simulink model "UR5_simulink"  (R2022b)
settings: Solver=FixedStepAuto  StartTime=0.0  StopTime=8  FixedStep=1e-4  RelTol=1e-3  AbsTol=1e-3  EnableMultiTasking=on
values from neighbouring files (symbols this model uses):
  a1 = 0    [UR5_matlab.m]
  a2 = -0.425    [UR5_matlab.m]
  a3 = -0.39225    [UR5_matlab.m]
  a4 = 0    [UR5_matlab.m]
  a5 = 0    [UR5_matlab.m]
  a6 = 0    [UR5_matlab.m]
  d1 = 0.089159    [UR5_matlab.m]
  d2 = 0    [UR5_matlab.m]
  d3 = 0    [UR5_matlab.m]
  d4 = 0.10915    [UR5_matlab.m]
  d5 = 0.09465    [UR5_matlab.m]
  d6 = 0.0823    [UR5_matlab.m]
  K_fb_1 = fb_action(K1_20,N,Jin_20,Bmw,J1_est,wR1)    [UR5_matlab.m]
  K_fb_2 = fb_action(K1_20,N,Jin_20,Bmw,J2_est,wR2)    [UR5_matlab.m]
  K_fb_3 = fb_action(K1_20,N,Jin_20,Bmw,J3_est,wR3)    [UR5_matlab.m]
  K_fb_4 = fb_action(K1_14,N,Jin_14,Bmw,J4_est,wR4)    [UR5_matlab.m]
  K_fb_5 = fb_action(K1_14,N,Jin_14,Bmw,J5_est,wR5)    [UR5_matlab.m]
  K_fb_6 = fb_action(K1_14,N,Jin_14,Bmw,J6_est,wR6)    [UR5_matlab.m]
  m1 = 3.7    [UR5_matlab.m]
  m2 = 8.393    [UR5_matlab.m]
  m3 = 2.33    [UR5_matlab.m]
  m4 = 1.1219    [UR5_matlab.m]
  m5 = 1.1219    [UR5_matlab.m]
  m6 = 0.1879    [UR5_matlab.m]
  N = 100    [UR5_matlab.m]
undefined symbols (not defined in the file or in its folder): X, Y, Z
libraries: fl_lib x60, sm_lib x33, nesl_utility x31, MyComponent_lib x12
(part 2 of 2)

== system UR5_simulink/Joint 1 ==
  PS-Simulink Converter1 : nesl_utility/PS-Simulink Converter  PhysicalDomain=network_engine_domain  SubClassName=ps_output  LeftPortType=input  RightPortType=output  PseudoPeriodic=off  Frequencies=[]  VectorFormat=1-D array  Unit=inherit  AffineConversion=off
  PS-Simulink Converter2 : nesl_utility/PS-Simulink Converter  PhysicalDomain=network_engine_domain  SubClassName=ps_output  LeftPortType=input  RightPortType=output  PseudoPeriodic=off  Frequencies=[]  VectorFormat=1-D array  Unit=inherit  AffineConversion=off
  R(x1,apha1) : sm_lib/Frames and Transforms/Rigid Transform  TranslationMethod=None  TranslationStandardOffset=0  TranslationLengthUnit=m  TranslationStandardAxis=+Z  TranslationCartesianOffset=[0 0 0]  TranslationROffset=0  TranslationROffsetUnits=m  TranslationZOffset=0  TranslationZOffsetUnits=m  TranslationThetaOffset=0  TranslationThetaOffsetUnits=deg  RotationMethod=StandardAxis  RotationAngleUnits=deg  RotationStandardAxis=+X  RotationAngle=alpha1  RotationArbitraryAxis=[0 0 1]  FollAlignAxisA=+X  BaseAlignAxisA=+Y  FollAlignAxisB=+Y  BaseAlignAxisB=+Z  RotationSequenceAxes=FollowerAxes  RotationSequence=XYX  RotationSequenceAngles=[0 0 0]  RotationSequenceAnglesUnits=deg  RotationMatrix=|  Quaternion=[1 0 0 0]
      | [1 0 0; 0 0 -1;
      | 0 1 0]
  R(zo,q1) : sm_lib/Joints/Revolute Joint  JointMode=Normal  SenseConstraintForce=off  SenseConstraintForceX=off  SenseConstraintForceY=off  SenseConstraintForceZ=off  SenseConstraintTorque=off  SenseConstraintTorqueX=off  SenseConstraintTorqueY=off  SenseConstraintTorqueZ=off  SenseTotalForce=off  SenseTotalForceX=off  SenseTotalForceY=off  SenseTotalForceZ=off  SenseTotalTorque=off  SenseTotalTorqueX=off  SenseTotalTorqueY=off  SenseTotalTorqueZ=off  CompositeWrenchDir=FollowerOnBase  CompositeWrenchFrame=BaseFrame  EquilibriumPosition=0  EquilibriumPositionUnits=deg  SpringStiffness=0  SpringStiffnessUnits=N*m/deg  DampingCoefficient=0  DampingCoefficientUnits=N*m/(deg/s)  TorqueActuationMode=InputTorque  MotionActuationMode=ComputedMotion  SensePosition=on  SenseVelocity=on  SenseAcceleration=off  SenseTorqueForce=off  SenseLowerLimitTorqueForce=off  SenseUpperLimitTorqueForce=off  LowerLimitSpecify=off  LowerLimitBound=-90  LowerLimitBoundUnits=deg  LowerLimitStiffness=1e4  LowerLimitStiffnessUnits=N*m/deg  LowerLimitDamping=10  LowerLimitDampingUnits=N*m/(deg/s)  LowerLimitTransitionRegionWidth=0.1  LowerLimitTransitionRegionWidthUnits=deg  UpperLimitSpecify=off  UpperLimitBound=90  UpperLimitBoundUnits=deg  UpperLimitStiffness=1e4  UpperLimitStiffnessUnits=N*m/deg  UpperLimitDamping=10  UpperLimitDampingUnits=N*m/(deg/s)  UpperLimitTransitionRegionWidth=0.1  UpperLimitTransitionRegionWidthUnits=deg  PositionTargetSpecify=off  PositionTargetPriority=High  PositionTargetValue=0  PositionTargetValueUnits=deg  VelocityTargetSpecify=off  VelocityTargetPriority=High  VelocityTargetValue=0  VelocityTargetValueUnits=deg/s
  T(x1,a1) : sm_lib/Frames and Transforms/Rigid Transform  TranslationMethod=Cartesian  TranslationStandardOffset=0  TranslationLengthUnit=m  TranslationStandardAxis=+X  TranslationCartesianOffset=[a1 0 0]  TranslationROffset=0  TranslationROffsetUnits=m  TranslationZOffset=0  TranslationZOffsetUnits=m  TranslationThetaOffset=0  TranslationThetaOffsetUnits=deg  RotationMethod=None  RotationAngleUnits=deg  RotationStandardAxis=+Z  RotationAngle=0.0  RotationArbitraryAxis=[0 0 1]  FollAlignAxisA=+X  BaseAlignAxisA=+Y  FollAlignAxisB=+Y  BaseAlignAxisB=+Z  RotationSequenceAxes=FollowerAxes  RotationSequence=XYX  RotationSequenceAngles=[0 0 0]  RotationSequenceAnglesUnits=deg  RotationMatrix=[1 0 0; 0 1 0; 0 0 1]  Quaternion=[1 0 0 0]
  T(z0,d1) : sm_lib/Frames and Transforms/Rigid Transform  TranslationMethod=Cartesian  TranslationStandardOffset=0.089159  TranslationLengthUnit=m  TranslationStandardAxis=+Z  TranslationCartesianOffset=[0 0 d1]  TranslationROffset=0  TranslationROffsetUnits=m  TranslationZOffset=0  TranslationZOffsetUnits=m  TranslationThetaOffset=0  TranslationThetaOffsetUnits=deg  RotationMethod=None  RotationAngleUnits=deg  RotationStandardAxis=+Z  RotationAngle=0.0  RotationArbitraryAxis=[0 0 1]  FollAlignAxisA=+X  BaseAlignAxisA=+Y  FollAlignAxisB=+Y  BaseAlignAxisB=+Z  RotationSequenceAxes=FollowerAxes  RotationSequence=XYX  RotationSequenceAngles=[0 0 0]  RotationSequenceAnglesUnits=deg  RotationMatrix=[1 0 0; 0 1 0; 0 0 1]  Quaternion=[1 0 0 0]
  Link 0 : PMIOPort  Side=Left
  Link 1 : PMIOPort  Port=2  Side=Right
  Joint velocity : PMIOPort  Port=3  Side=Right
  Joint torque1 : PMIOPort  Port=4  Side=Left
  tag scope: dq1=global, q1=global
  wires:
  PS-Simulink Converter1/1 -> [q1]
  PS-Simulink Converter2/1 -> [dq1]
  connections:
  PS-Simulink Converter2/LConn1 -- R(zo,q1)/RConn3 -- Joint velocity/RConn1
  PS-Simulink Converter1/LConn1 -- R(zo,q1)/RConn2
  T(z0,d1)/LConn1 -- Link 0/RConn1
  R(zo,q1)/LConn1 -- T(z0,d1)/RConn1
  T(x1,a1)/LConn1 -- R(zo,q1)/RConn1
  Joint torque1/RConn1 -- R(zo,q1)/LConn2
  R(x1,apha1)/LConn1 -- T(x1,a1)/RConn1
  R(x1,apha1)/RConn1 -- Link 1/RConn1

== system UR5_simulink/Joint 2 ==
  PS-Simulink Converter1 : nesl_utility/PS-Simulink Converter  PhysicalDomain=network_engine_domain  SubClassName=ps_output  LeftPortType=input  RightPortType=output  PseudoPeriodic=off  Frequencies=[]  VectorFormat=1-D array  Unit=inherit  AffineConversion=off
  PS-Simulink Converter2 : nesl_utility/PS-Simulink Converter  PhysicalDomain=network_engine_domain  SubClassName=ps_output  LeftPortType=input  RightPortType=output  PseudoPeriodic=off  Frequencies=[]  VectorFormat=1-D array  Unit=inherit  AffineConversion=off
  R(x2,alpha2) : sm_lib/Frames and Transforms/Rigid Transform  TranslationMethod=None  TranslationStandardOffset=0  TranslationLengthUnit=m  TranslationStandardAxis=+Z  TranslationCartesianOffset=[-0.425 0 0]  TranslationROffset=0  TranslationROffsetUnits=m  TranslationZOffset=0  TranslationZOffsetUnits=m  TranslationThetaOffset=0  TranslationThetaOffsetUnits=deg  RotationMethod=StandardAxis  RotationAngleUnits=deg  RotationStandardAxis=+X  RotationAngle=alpha2  RotationArbitraryAxis=[0 0 1]  FollAlignAxisA=+X  BaseAlignAxisA=+Y  FollAlignAxisB=+Y  BaseAlignAxisB=+Z  RotationSequenceAxes=FollowerAxes  RotationSequence=XYX  RotationSequenceAngles=[0 0 0]  RotationSequenceAnglesUnits=deg  RotationMatrix=[1 0 0; 0 1 0; 0 0 1]  Quaternion=[1 0 0 0]
  R(z1,q2) : sm_lib/Joints/Revolute Joint  JointMode=Normal  SenseConstraintForce=off  SenseConstraintForceX=off  SenseConstraintForceY=off  SenseConstraintForceZ=off  SenseConstraintTorque=off  SenseConstraintTorqueX=off  SenseConstraintTorqueY=off  SenseConstraintTorqueZ=off  SenseTotalForce=off  SenseTotalForceX=off  SenseTotalForceY=off  SenseTotalForceZ=off  SenseTotalTorque=off  SenseTotalTorqueX=off  SenseTotalTorqueY=off  SenseTotalTorqueZ=off  CompositeWrenchDir=FollowerOnBase  CompositeWrenchFrame=BaseFrame  EquilibriumPosition=0  EquilibriumPositionUnits=deg  SpringStiffness=0  SpringStiffnessUnits=N*m/deg  DampingCoefficient=0  DampingCoefficientUnits=N*m/(deg/s)  TorqueActuationMode=InputTorque  MotionActuationMode=ComputedMotion  SensePosition=on  SenseVelocity=on  SenseAcceleration=off  SenseTorqueForce=off  SenseLowerLimitTorqueForce=off  SenseUpperLimitTorqueForce=off  LowerLimitSpecify=off  LowerLimitBound=-360  LowerLimitBoundUnits=deg  LowerLimitStiffness=1e4  LowerLimitStiffnessUnits=N*m/deg  LowerLimitDamping=10  LowerLimitDampingUnits=N*m/(deg/s)  LowerLimitTransitionRegionWidth=0.1  LowerLimitTransitionRegionWidthUnits=deg  UpperLimitSpecify=off  UpperLimitBound=360  UpperLimitBoundUnits=deg  UpperLimitStiffness=1e4  UpperLimitStiffnessUnits=N*m/deg  UpperLimitDamping=10  UpperLimitDampingUnits=N*m/(deg/s)  UpperLimitTransitionRegionWidth=0.1  UpperLimitTransitionRegionWidthUnits=deg  PositionTargetSpecify=off  PositionTargetPriority=High  PositionTargetValue=0  PositionTargetValueUnits=deg  VelocityTargetSpecify=off  VelocityTargetPriority=High  VelocityTargetValue=0  VelocityTargetValueUnits=deg/s
  T(x2,a2) : sm_lib/Frames and Transforms/Rigid Transform  TranslationMethod=Cartesian  TranslationStandardOffset=0.425  TranslationLengthUnit=m  TranslationStandardAxis=-X  TranslationCartesianOffset=[a2 0 0]  TranslationROffset=0  TranslationROffsetUnits=m  TranslationZOffset=0  TranslationZOffsetUnits=m  TranslationThetaOffset=0  TranslationThetaOffsetUnits=deg  RotationMethod=None  RotationAngleUnits=deg  RotationStandardAxis=+Z  RotationAngle=0.0  RotationArbitraryAxis=[0 0 1]  FollAlignAxisA=+X  BaseAlignAxisA=+Y  FollAlignAxisB=+Y  BaseAlignAxisB=+Z  RotationSequenceAxes=FollowerAxes  RotationSequence=XYX  RotationSequenceAngles=[0 0 0]  RotationSequenceAnglesUnits=deg  RotationMatrix=[1 0 0; 0 1 0; 0 0 1]  Quaternion=[1 0 0 0]
  T(z1,d2) : sm_lib/Frames and Transforms/Rigid Transform  TranslationMethod=Cartesian  TranslationStandardOffset=0  TranslationLengthUnit=m  TranslationStandardAxis=+Z  TranslationCartesianOffset=[0 0 d2]  TranslationROffset=0  TranslationROffsetUnits=m  TranslationZOffset=0  TranslationZOffsetUnits=m  TranslationThetaOffset=0  TranslationThetaOffsetUnits=deg  RotationMethod=None  RotationAngleUnits=deg  RotationStandardAxis=+Z  RotationAngle=0.0  RotationArbitraryAxis=[0 0 1]  FollAlignAxisA=+X  BaseAlignAxisA=+Y  FollAlignAxisB=+Y  BaseAlignAxisB=+Z  RotationSequenceAxes=FollowerAxes  RotationSequence=XYX  RotationSequenceAngles=[0 0 0]  RotationSequenceAnglesUnits=deg  RotationMatrix=[1 -0 0; 0 1 0; 0 0 1]  Quaternion=[1 0 0 0]
  Link 1 : PMIOPort  Side=Left
  "Joint torque " : PMIOPort  Port=2  Side=Left
  Link 2 : PMIOPort  Port=3  Side=Right
  Joint velocity : PMIOPort  Port=4  Side=Right
  tag scope: dq2=global, q2=global
  wires:
  PS-Simulink Converter2/1 -> [dq2]
  PS-Simulink Converter1/1 -> [q2]
  connections:
  R(z1,q2)/LConn1 -- T(z1,d2)/RConn1
  PS-Simulink Converter2/LConn1 -- R(z1,q2)/RConn3 -- Joint velocity/RConn1
  PS-Simulink Converter1/LConn1 -- R(z1,q2)/RConn2
  T(z1,d2)/LConn1 -- Link 1/RConn1
  T(x2,a2)/LConn1 -- R(z1,q2)/RConn1
  "Joint torque "/RConn1 -- R(z1,q2)/LConn2
  R(x2,alpha2)/LConn1 -- T(x2,a2)/RConn1
  Link 2/RConn1 -- R(x2,alpha2)/RConn1

== system UR5_simulink/Joint 3 ==
  PS-Simulink Converter1 : nesl_utility/PS-Simulink Converter  PhysicalDomain=network_engine_domain  SubClassName=ps_output  LeftPortType=input  RightPortType=output  PseudoPeriodic=off  Frequencies=[]  VectorFormat=1-D array  Unit=inherit  AffineConversion=off
  PS-Simulink Converter2 : nesl_utility/PS-Simulink Converter  PhysicalDomain=network_engine_domain  SubClassName=ps_output  LeftPortType=input  RightPortType=output  PseudoPeriodic=off  Frequencies=[]  VectorFormat=1-D array  Unit=inherit  AffineConversion=off
  R(x3,alpha3) : sm_lib/Frames and Transforms/Rigid Transform  TranslationMethod=None  TranslationStandardOffset=0  TranslationLengthUnit=m  TranslationStandardAxis=+Z  TranslationCartesianOffset=[-0.425 0 0]  TranslationROffset=0  TranslationROffsetUnits=m  TranslationZOffset=0  TranslationZOffsetUnits=m  TranslationThetaOffset=0  TranslationThetaOffsetUnits=deg  RotationMethod=StandardAxis  RotationAngleUnits=deg  RotationStandardAxis=+X  RotationAngle=alpha3  RotationArbitraryAxis=[0 0 1]  FollAlignAxisA=+X  BaseAlignAxisA=+Y  FollAlignAxisB=+Y  BaseAlignAxisB=+Z  RotationSequenceAxes=FollowerAxes  RotationSequence=XYX  RotationSequenceAngles=[0 0 0]  RotationSequenceAnglesUnits=deg  RotationMatrix=[1 0 0; 0 1 0; 0 0 1]  Quaternion=[1 0 0 0]
  R(z2,q3) : sm_lib/Joints/Revolute Joint  JointMode=Normal  SenseConstraintForce=off  SenseConstraintForceX=off  SenseConstraintForceY=off  SenseConstraintForceZ=off  SenseConstraintTorque=off  SenseConstraintTorqueX=off  SenseConstraintTorqueY=off  SenseConstraintTorqueZ=off  SenseTotalForce=off  SenseTotalForceX=off  SenseTotalForceY=off  SenseTotalForceZ=off  SenseTotalTorque=off  SenseTotalTorqueX=off  SenseTotalTorqueY=off  SenseTotalTorqueZ=off  CompositeWrenchDir=FollowerOnBase  CompositeWrenchFrame=BaseFrame  EquilibriumPosition=0  EquilibriumPositionUnits=deg  SpringStiffness=0  SpringStiffnessUnits=N*m/deg  DampingCoefficient=0  DampingCoefficientUnits=N*m/(deg/s)  TorqueActuationMode=InputTorque  MotionActuationMode=ComputedMotion  SensePosition=on  SenseVelocity=on  SenseAcceleration=off  SenseTorqueForce=off  SenseLowerLimitTorqueForce=off  SenseUpperLimitTorqueForce=off  LowerLimitSpecify=off  LowerLimitBound=-360  LowerLimitBoundUnits=deg  LowerLimitStiffness=1e4  LowerLimitStiffnessUnits=N*m/deg  LowerLimitDamping=10  LowerLimitDampingUnits=N*m/(deg/s)  LowerLimitTransitionRegionWidth=0.1  LowerLimitTransitionRegionWidthUnits=deg  UpperLimitSpecify=off  UpperLimitBound=360  UpperLimitBoundUnits=deg  UpperLimitStiffness=1e4  UpperLimitStiffnessUnits=N*m/deg  UpperLimitDamping=10  UpperLimitDampingUnits=N*m/(deg/s)  UpperLimitTransitionRegionWidth=0.1  UpperLimitTransitionRegionWidthUnits=deg  PositionTargetSpecify=off  PositionTargetPriority=High  PositionTargetValue=0  PositionTargetValueUnits=deg  VelocityTargetSpecify=off  VelocityTargetPriority=High  VelocityTargetValue=0  VelocityTargetValueUnits=deg/s
  T(x3,a3) : sm_lib/Frames and Transforms/Rigid Transform  TranslationMethod=Cartesian  TranslationStandardOffset=-0.39225  TranslationLengthUnit=m  TranslationStandardAxis=+X  TranslationCartesianOffset=[a3 0 0]  TranslationROffset=0  TranslationROffsetUnits=m  TranslationZOffset=0  TranslationZOffsetUnits=m  TranslationThetaOffset=0  TranslationThetaOffsetUnits=deg  RotationMethod=None  RotationAngleUnits=deg  RotationStandardAxis=+Z  RotationAngle=0.0  RotationArbitraryAxis=[0 0 1]  FollAlignAxisA=+X  BaseAlignAxisA=+Y  FollAlignAxisB=+Y  BaseAlignAxisB=+Z  RotationSequenceAxes=FollowerAxes  RotationSequence=XYX  RotationSequenceAngles=[0 0 0]  RotationSequenceAnglesUnits=deg  RotationMatrix=[1 0 0; 0 1 0; 0 0 1]  Quaternion=[1 0 0 0]
  T(z2,d3) : sm_lib/Frames and Transforms/Rigid Transform  TranslationMethod=Cartesian  TranslationStandardOffset=0  TranslationLengthUnit=m  TranslationStandardAxis=+Z  TranslationCartesianOffset=[0 0 d3]  TranslationROffset=0  TranslationROffsetUnits=m  TranslationZOffset=0  TranslationZOffsetUnits=m  TranslationThetaOffset=0  TranslationThetaOffsetUnits=deg  RotationMethod=None  RotationAngleUnits=deg  RotationStandardAxis=+Z  RotationAngle=0.0  RotationArbitraryAxis=[0 0 1]  FollAlignAxisA=+X  BaseAlignAxisA=+Y  FollAlignAxisB=+Y  BaseAlignAxisB=+Z  RotationSequenceAxes=FollowerAxes  RotationSequence=XYX  RotationSequenceAngles=[0 0 0]  RotationSequenceAnglesUnits=deg  RotationMatrix=[1 -0 0; 0 1 0; 0 0 1]  Quaternion=[1 0 0 0]
  Link 2 : PMIOPort  Side=Left
  "Joint torque " : PMIOPort  Port=2  Side=Left
  Link 3 : PMIOPort  Port=3  Side=Right
  Joint velocity : PMIOPort  Port=4  Side=Right
  tag scope: dq3=global, q3=global
  wires:
  PS-Simulink Converter2/1 -> [dq3]
  PS-Simulink Converter1/1 -> [q3]
  connections:
  PS-Simulink Converter2/LConn1 -- Joint velocity/RConn1 -- R(z2,q3)/RConn3
  PS-Simulink Converter1/LConn1 -- R(z2,q3)/RConn2
  T(z2,d3)/RConn1 -- R(z2,q3)/LConn1
  T(z2,d3)/LConn1 -- Link 2/RConn1
  T(x3,a3)/LConn1 -- R(z2,q3)/RConn1
  R(z2,q3)/LConn2 -- "Joint torque "/RConn1
  R(x3,alpha3)/RConn1 -- Link 3/RConn1
  T(x3,a3)/RConn1 -- R(x3,alpha3)/LConn1

== system UR5_simulink/Joint 4 ==
  PS-Simulink Converter1 : nesl_utility/PS-Simulink Converter  PhysicalDomain=network_engine_domain  SubClassName=ps_output  LeftPortType=input  RightPortType=output  PseudoPeriodic=off  Frequencies=[]  VectorFormat=1-D array  Unit=inherit  AffineConversion=off
  PS-Simulink Converter2 : nesl_utility/PS-Simulink Converter  PhysicalDomain=network_engine_domain  SubClassName=ps_output  LeftPortType=input  RightPortType=output  PseudoPeriodic=off  Frequencies=[]  VectorFormat=1-D array  Unit=inherit  AffineConversion=off
  R(x4,alpha4) : sm_lib/Frames and Transforms/Rigid Transform  TranslationMethod=None  TranslationStandardOffset=0  TranslationLengthUnit=m  TranslationStandardAxis=+Z  TranslationCartesianOffset=[0 0 0]  TranslationROffset=0  TranslationROffsetUnits=m  TranslationZOffset=0  TranslationZOffsetUnits=m  TranslationThetaOffset=0  TranslationThetaOffsetUnits=deg  RotationMethod=StandardAxis  RotationAngleUnits=deg  RotationStandardAxis=+X  RotationAngle=alpha4  RotationArbitraryAxis=[0 0 1]  FollAlignAxisA=+X  BaseAlignAxisA=+Y  FollAlignAxisB=+Y  BaseAlignAxisB=+Z  RotationSequenceAxes=FollowerAxes  RotationSequence=XYX  RotationSequenceAngles=[0 0 0]  RotationSequenceAnglesUnits=deg  RotationMatrix=[1 0 0; 0 1 0; 0 0 1]  Quaternion=[1 0 0 0]
  R(z3,q4) : sm_lib/Joints/Revolute Joint  JointMode=Normal  SenseConstraintForce=off  SenseConstraintForceX=off  SenseConstraintForceY=off  SenseConstraintForceZ=off  SenseConstraintTorque=off  SenseConstraintTorqueX=off  SenseConstraintTorqueY=off  SenseConstraintTorqueZ=off  SenseTotalForce=off  SenseTotalForceX=off  SenseTotalForceY=off  SenseTotalForceZ=off  SenseTotalTorque=off  SenseTotalTorqueX=off  SenseTotalTorqueY=off  SenseTotalTorqueZ=off  CompositeWrenchDir=FollowerOnBase  CompositeWrenchFrame=BaseFrame  EquilibriumPosition=0  EquilibriumPositionUnits=deg  SpringStiffness=0  SpringStiffnessUnits=N*m/deg  DampingCoefficient=Bmw  DampingCoefficientUnits=N*m/(deg/s)  TorqueActuationMode=InputTorque  MotionActuationMode=ComputedMotion  SensePosition=on  SenseVelocity=on  SenseAcceleration=off  SenseTorqueForce=off  SenseLowerLimitTorqueForce=off  SenseUpperLimitTorqueForce=off  LowerLimitSpecify=off  LowerLimitBound=-360  LowerLimitBoundUnits=deg  LowerLimitStiffness=1e4  LowerLimitStiffnessUnits=N*m/deg  LowerLimitDamping=10  LowerLimitDampingUnits=N*m/(deg/s)  LowerLimitTransitionRegionWidth=0.1  LowerLimitTransitionRegionWidthUnits=deg  UpperLimitSpecify=off  UpperLimitBound=360  UpperLimitBoundUnits=deg  UpperLimitStiffness=1e4  UpperLimitStiffnessUnits=N*m/deg  UpperLimitDamping=10  UpperLimitDampingUnits=N*m/(deg/s)  UpperLimitTransitionRegionWidth=0.1  UpperLimitTransitionRegionWidthUnits=deg  PositionTargetSpecify=off  PositionTargetPriority=High  PositionTargetValue=0  PositionTargetValueUnits=deg  VelocityTargetSpecify=off  VelocityTargetPriority=High  VelocityTargetValue=0  VelocityTargetValueUnits=deg/s
  T(x4,a4) : sm_lib/Frames and Transforms/Rigid Transform  TranslationMethod=Cartesian  TranslationStandardOffset=0  TranslationLengthUnit=m  TranslationStandardAxis=+X  TranslationCartesianOffset=[a4 0 0]  TranslationROffset=0  TranslationROffsetUnits=m  TranslationZOffset=0  TranslationZOffsetUnits=m  TranslationThetaOffset=0  TranslationThetaOffsetUnits=deg  RotationMethod=None  RotationAngleUnits=deg  RotationStandardAxis=+Z  RotationAngle=0.0  RotationArbitraryAxis=[0 0 1]  FollAlignAxisA=+X  BaseAlignAxisA=+Y  FollAlignAxisB=+Y  BaseAlignAxisB=+Z  RotationSequenceAxes=FollowerAxes  RotationSequence=XYX  RotationSequenceAngles=[0 0 0]  RotationSequenceAnglesUnits=deg  RotationMatrix=[1 0 0; 0 1 0; 0 0 1]  Quaternion=[1 0 0 0]
  T(z3,d4) : sm_lib/Frames and Transforms/Rigid Transform  TranslationMethod=Cartesian  TranslationStandardOffset=0.10915  TranslationLengthUnit=m  TranslationStandardAxis=+Z  TranslationCartesianOffset=[0 0 d4]  TranslationROffset=0  TranslationROffsetUnits=m  TranslationZOffset=0  TranslationZOffsetUnits=m  TranslationThetaOffset=0  TranslationThetaOffsetUnits=deg  RotationMethod=None  RotationAngleUnits=deg  RotationStandardAxis=+Z  RotationAngle=0.0  RotationArbitraryAxis=[0 0 1]  FollAlignAxisA=+X  BaseAlignAxisA=+Y  FollAlignAxisB=+Y  BaseAlignAxisB=+Z  RotationSequenceAxes=FollowerAxes  RotationSequence=XYX  RotationSequenceAngles=[0 0 0]  RotationSequenceAnglesUnits=deg  RotationMatrix=[1 0 0; 0 1 0; 0 0 1]  Quaternion=[1 0 0 0]
  Link 3 : PMIOPort  Side=Left
  "Joint torque " : PMIOPort  Port=2  Side=Left
  Link 4 : PMIOPort  Port=3  Side=Right
  Joint velocity : PMIOPort  Port=4  Side=Right
  tag scope: dq4=global, q4=global
  wires:
  PS-Simulink Converter1/1 -> [q4]
  PS-Simulink Converter2/1 -> [dq4]
  connections:
  Link 3/RConn1 -- T(z3,d4)/LConn1
  PS-Simulink Converter2/LConn1 -- Joint velocity/RConn1 -- R(z3,q4)/RConn3
  PS-Simulink Converter1/LConn1 -- R(z3,q4)/RConn2
  T(z3,d4)/RConn1 -- R(z3,q4)/LConn1
  T(x4,a4)/LConn1 -- R(z3,q4)/RConn1
  R(z3,q4)/LConn2 -- "Joint torque "/RConn1
  R(x4,alpha4)/LConn1 -- T(x4,a4)/RConn1
  Link 4/RConn1 -- R(x4,alpha4)/RConn1

== system UR5_simulink/Joint 5 ==
  PS-Simulink Converter1 : nesl_utility/PS-Simulink Converter  PhysicalDomain=network_engine_domain  SubClassName=ps_output  LeftPortType=input  RightPortType=output  PseudoPeriodic=off  Frequencies=[]  VectorFormat=1-D array  Unit=inherit  AffineConversion=off
  PS-Simulink Converter2 : nesl_utility/PS-Simulink Converter  PhysicalDomain=network_engine_domain  SubClassName=ps_output  LeftPortType=input  RightPortType=output  PseudoPeriodic=off  Frequencies=[]  VectorFormat=1-D array  Unit=inherit  AffineConversion=off
  R(x5,alpha5) : sm_lib/Frames and Transforms/Rigid Transform  TranslationMethod=None  TranslationStandardOffset=0  TranslationLengthUnit=m  TranslationStandardAxis=+Z  TranslationCartesianOffset=[0 0 0]  TranslationROffset=0  TranslationROffsetUnits=m  TranslationZOffset=0  TranslationZOffsetUnits=m  TranslationThetaOffset=0  TranslationThetaOffsetUnits=deg  RotationMethod=StandardAxis  RotationAngleUnits=deg  RotationStandardAxis=+X  RotationAngle=alpha5  RotationArbitraryAxis=[0 0 1]  FollAlignAxisA=+X  BaseAlignAxisA=+Y  FollAlignAxisB=+Y  BaseAlignAxisB=+Z  RotationSequenceAxes=FollowerAxes  RotationSequence=XYX  RotationSequenceAngles=[0 0 0]  RotationSequenceAnglesUnits=deg  RotationMatrix=[1 0 0; 0 1 0; 0 0 1]  Quaternion=[1 0 0 0]
  R(z4,q5) : sm_lib/Joints/Revolute Joint  JointMode=Normal  SenseConstraintForce=off  SenseConstraintForceX=off  SenseConstraintForceY=off  SenseConstraintForceZ=off  SenseConstraintTorque=off  SenseConstraintTorqueX=off  SenseConstraintTorqueY=off  SenseConstraintTorqueZ=off  SenseTotalForce=off  SenseTotalForceX=off  SenseTotalForceY=off  SenseTotalForceZ=off  SenseTotalTorque=off  SenseTotalTorqueX=off  SenseTotalTorqueY=off  SenseTotalTorqueZ=off  CompositeWrenchDir=FollowerOnBase  CompositeWrenchFrame=BaseFrame  EquilibriumPosition=0  EquilibriumPositionUnits=deg  SpringStiffness=0  SpringStiffnessUnits=N*m/deg  DampingCoefficient=Bmw  DampingCoefficientUnits=N*m/(deg/s)  TorqueActuationMode=InputTorque  MotionActuationMode=ComputedMotion  SensePosition=on  SenseVelocity=on  SenseAcceleration=off  SenseTorqueForce=off  SenseLowerLimitTorqueForce=off  SenseUpperLimitTorqueForce=off  LowerLimitSpecify=off  LowerLimitBound=-360  LowerLimitBoundUnits=deg  LowerLimitStiffness=1e4  LowerLimitStiffnessUnits=N*m/deg  LowerLimitDamping=10  LowerLimitDampingUnits=N*m/(deg/s)  LowerLimitTransitionRegionWidth=0.1  LowerLimitTransitionRegionWidthUnits=deg  UpperLimitSpecify=off  UpperLimitBound=360  UpperLimitBoundUnits=deg  UpperLimitStiffness=1e4  UpperLimitStiffnessUnits=N*m/deg  UpperLimitDamping=10  UpperLimitDampingUnits=N*m/(deg/s)  UpperLimitTransitionRegionWidth=0.1  UpperLimitTransitionRegionWidthUnits=deg  PositionTargetSpecify=off  PositionTargetPriority=High  PositionTargetValue=0  PositionTargetValueUnits=deg  VelocityTargetSpecify=off  VelocityTargetPriority=High  VelocityTargetValue=0  VelocityTargetValueUnits=deg/s
  T(x5,a5) : sm_lib/Frames and Transforms/Rigid Transform  TranslationMethod=Cartesian  TranslationStandardOffset=0  TranslationLengthUnit=m  TranslationStandardAxis=+X  TranslationCartesianOffset=[a5 0 0]  TranslationROffset=0  TranslationROffsetUnits=m  TranslationZOffset=0  TranslationZOffsetUnits=m  TranslationThetaOffset=0  TranslationThetaOffsetUnits=deg  RotationMethod=None  RotationAngleUnits=deg  RotationStandardAxis=+Z  RotationAngle=0.0  RotationArbitraryAxis=[0 0 1]  FollAlignAxisA=+X  BaseAlignAxisA=+Y  FollAlignAxisB=+Y  BaseAlignAxisB=+Z  RotationSequenceAxes=FollowerAxes  RotationSequence=XYX  RotationSequenceAngles=[0 0 0]  RotationSequenceAnglesUnits=deg  RotationMatrix=[1 0 0; 0 1 0; 0 0 1]  Quaternion=[1 0 0 0]
  T(z4,d5) : sm_lib/Frames and Transforms/Rigid Transform  TranslationMethod=Cartesian  TranslationStandardOffset=0.09465  TranslationLengthUnit=m  TranslationStandardAxis=+Z  TranslationCartesianOffset=[0 0 d5]  TranslationROffset=0  TranslationROffsetUnits=m  TranslationZOffset=0  TranslationZOffsetUnits=m  TranslationThetaOffset=0  TranslationThetaOffsetUnits=deg  RotationMethod=None  RotationAngleUnits=deg  RotationStandardAxis=+Z  RotationAngle=0.0  RotationArbitraryAxis=[0 0 1]  FollAlignAxisA=+X  BaseAlignAxisA=+Y  FollAlignAxisB=+Y  BaseAlignAxisB=+Z  RotationSequenceAxes=FollowerAxes  RotationSequence=XYX  RotationSequenceAngles=[0 0 0]  RotationSequenceAnglesUnits=deg  RotationMatrix=[1 0 0; 0 1 0; 0 0 1]  Quaternion=[1 0 0 0]
  "Joint torque " : PMIOPort  Side=Left
  Link 4 : PMIOPort  Port=2  Side=Left
  Joint velocity : PMIOPort  Port=3  Side=Right
  Link 5 : PMIOPort  Port=4  Side=Right
  tag scope: dq5=global, q5=global
  wires:
  PS-Simulink Converter2/1 -> [dq5]
  PS-Simulink Converter1/1 -> [q5]
  connections:
  Link 4/RConn1 -- T(z4,d5)/LConn1
  PS-Simulink Converter2/LConn1 -- R(z4,q5)/RConn3 -- Joint velocity/RConn1
  PS-Simulink Converter1/LConn1 -- R(z4,q5)/RConn2
  T(z4,d5)/RConn1 -- R(z4,q5)/LConn1
  T(x5,a5)/LConn1 -- R(z4,q5)/RConn1
  "Joint torque "/RConn1 -- R(z4,q5)/LConn2
  R(x5,alpha5)/LConn1 -- T(x5,a5)/RConn1
  Link 5/RConn1 -- R(x5,alpha5)/RConn1

== system UR5_simulink/Joint 6 ==
  PS-Simulink Converter1 : nesl_utility/PS-Simulink Converter  PhysicalDomain=network_engine_domain  SubClassName=ps_output  LeftPortType=input  RightPortType=output  PseudoPeriodic=off  Frequencies=[]  VectorFormat=1-D array  Unit=inherit  AffineConversion=off
  PS-Simulink Converter2 : nesl_utility/PS-Simulink Converter  PhysicalDomain=network_engine_domain  SubClassName=ps_output  LeftPortType=input  RightPortType=output  PseudoPeriodic=off  Frequencies=[]  VectorFormat=1-D array  Unit=inherit  AffineConversion=off
  R(x6,alpha6) : sm_lib/Frames and Transforms/Rigid Transform  TranslationMethod=None  TranslationStandardOffset=0  TranslationLengthUnit=m  TranslationStandardAxis=+Z  TranslationCartesianOffset=[0 0 0]  TranslationROffset=0  TranslationROffsetUnits=m  TranslationZOffset=0  TranslationZOffsetUnits=m  TranslationThetaOffset=0  TranslationThetaOffsetUnits=deg  RotationMethod=StandardAxis  RotationAngleUnits=deg  RotationStandardAxis=+X  RotationAngle=alpha6  RotationArbitraryAxis=[0 0 1]  FollAlignAxisA=+X  BaseAlignAxisA=+Y  FollAlignAxisB=+Y  BaseAlignAxisB=+Z  RotationSequenceAxes=FollowerAxes  RotationSequence=XYX  RotationSequenceAngles=[0 0 0]  RotationSequenceAnglesUnits=deg  RotationMatrix=[1 0 0; 0 1 0; 0 0 1]  Quaternion=[1 0 0 0]
  R(z5,q6) : sm_lib/Joints/Revolute Joint  JointMode=Normal  SenseConstraintForce=off  SenseConstraintForceX=off  SenseConstraintForceY=off  SenseConstraintForceZ=off  SenseConstraintTorque=off  SenseConstraintTorqueX=off  SenseConstraintTorqueY=off  SenseConstraintTorqueZ=off  SenseTotalForce=off  SenseTotalForceX=off  SenseTotalForceY=off  SenseTotalForceZ=off  SenseTotalTorque=off  SenseTotalTorqueX=off  SenseTotalTorqueY=off  SenseTotalTorqueZ=off  CompositeWrenchDir=FollowerOnBase  CompositeWrenchFrame=BaseFrame  EquilibriumPosition=0  EquilibriumPositionUnits=deg  SpringStiffness=0  SpringStiffnessUnits=N*m/deg  DampingCoefficient=Bmw  DampingCoefficientUnits=N*m/(deg/s)  TorqueActuationMode=InputTorque  MotionActuationMode=ComputedMotion  SensePosition=on  SenseVelocity=on  SenseAcceleration=off  SenseTorqueForce=off  SenseLowerLimitTorqueForce=off  SenseUpperLimitTorqueForce=off  LowerLimitSpecify=off  LowerLimitBound=-360  LowerLimitBoundUnits=deg  LowerLimitStiffness=1e4  LowerLimitStiffnessUnits=N*m/deg  LowerLimitDamping=10  LowerLimitDampingUnits=N*m/(deg/s)  LowerLimitTransitionRegionWidth=0.1  LowerLimitTransitionRegionWidthUnits=deg  UpperLimitSpecify=off  UpperLimitBound=360  UpperLimitBoundUnits=deg  UpperLimitStiffness=1e4  UpperLimitStiffnessUnits=N*m/deg  UpperLimitDamping=10  UpperLimitDampingUnits=N*m/(deg/s)  UpperLimitTransitionRegionWidth=0.1  UpperLimitTransitionRegionWidthUnits=deg  PositionTargetSpecify=off  PositionTargetPriority=High  PositionTargetValue=0  PositionTargetValueUnits=deg  VelocityTargetSpecify=off  VelocityTargetPriority=High  VelocityTargetValue=0  VelocityTargetValueUnits=deg/s
  T(x6,a6) : sm_lib/Frames and Transforms/Rigid Transform  TranslationMethod=Cartesian  TranslationStandardOffset=0  TranslationLengthUnit=m  TranslationStandardAxis=+X  TranslationCartesianOffset=[a6 0 0]  TranslationROffset=0  TranslationROffsetUnits=m  TranslationZOffset=0  TranslationZOffsetUnits=m  TranslationThetaOffset=0  TranslationThetaOffsetUnits=deg  RotationMethod=None  RotationAngleUnits=deg  RotationStandardAxis=+Z  RotationAngle=0.0  RotationArbitraryAxis=[0 0 1]  FollAlignAxisA=+X  BaseAlignAxisA=+Y  FollAlignAxisB=+Y  BaseAlignAxisB=+Z  RotationSequenceAxes=FollowerAxes  RotationSequence=XYX  RotationSequenceAngles=[0 0 0]  RotationSequenceAnglesUnits=deg  RotationMatrix=[1 0 0; 0 1 0; 0 0 1]  Quaternion=[1 0 0 0]
  T(z5,d6) : sm_lib/Frames and Transforms/Rigid Transform  TranslationMethod=Cartesian  TranslationStandardOffset=0.0823  TranslationLengthUnit=m  TranslationStandardAxis=+Z  TranslationCartesianOffset=[0 0 d6]  TranslationROffset=0  TranslationROffsetUnits=m  TranslationZOffset=0  TranslationZOffsetUnits=m  TranslationThetaOffset=0  TranslationThetaOffsetUnits=deg  RotationMethod=None  RotationAngleUnits=deg  RotationStandardAxis=+Z  RotationAngle=0.0  RotationArbitraryAxis=[0 0 1]  FollAlignAxisA=+X  BaseAlignAxisA=+Y  FollAlignAxisB=+Y  BaseAlignAxisB=+Z  RotationSequenceAxes=FollowerAxes  RotationSequence=XYX  RotationSequenceAngles=[0 0 0]  RotationSequenceAnglesUnits=deg  RotationMatrix=[1 0 0; 0 1 0; 0 0 1]  Quaternion=[1 0 0 0]
  Link 5 : PMIOPort  Side=Left
  "Joint torque " : PMIOPort  Port=2  Side=Left
  Link 6 : PMIOPort  Port=3  Side=Right
  Joint velocity : PMIOPort  Port=4  Side=Right
  tag scope: dq6=global, q6=global
  wires:
  PS-Simulink Converter1/1 -> [q6]
  PS-Simulink Converter2/1 -> [dq6]
  connections:
  Link 5/RConn1 -- T(z5,d6)/LConn1
  Joint velocity/RConn1 -- PS-Simulink Converter2/LConn1 -- R(z5,q6)/RConn3
  PS-Simulink Converter1/LConn1 -- R(z5,q6)/RConn2
  T(z5,d6)/RConn1 -- R(z5,q6)/LConn1
  T(x6,a6)/LConn1 -- R(z5,q6)/RConn1
  "Joint torque "/RConn1 -- R(z5,q6)/LConn2
  R(x6,alpha6)/LConn1 -- T(x6,a6)/RConn1
  Link 6/RConn1 -- R(x6,alpha6)/RConn1

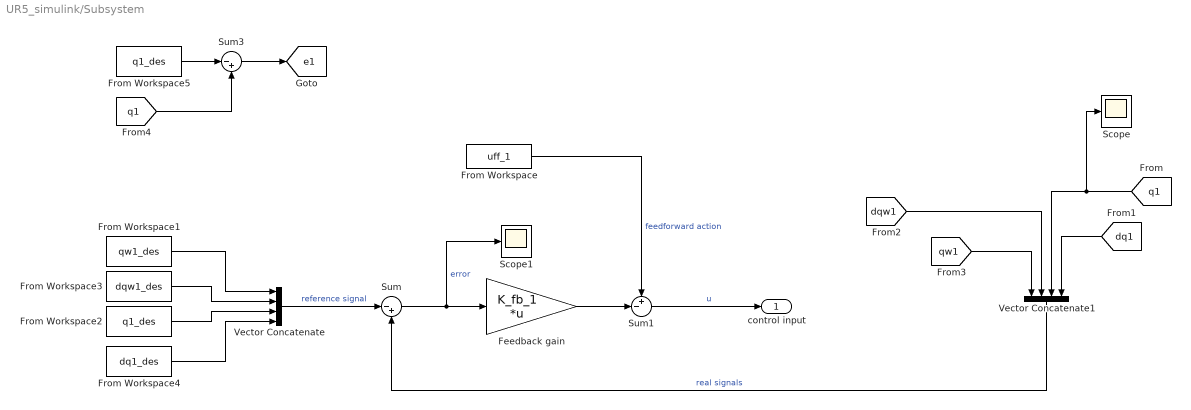
== system UR5_simulink/Subsystem ==
  Feedback gain : Gain  Gain=K_fb_1  Multiplication=Matrix(K*u) (u vector)
  From Workspace : FromWorkspace  VariableName=uff_1
  From Workspace1 : FromWorkspace  VariableName=qw1_des
  From Workspace2 : FromWorkspace  VariableName=q1_des
  From Workspace3 : FromWorkspace  VariableName=dqw1_des
  From Workspace4 : FromWorkspace  VariableName=dq1_des
  From Workspace5 : FromWorkspace  VariableName=q1_des
  Scope : Scope
  Scope1 : Scope
  Sum : Sum  Inputs=|-+
  Sum1 : Sum  Inputs=+-|
  Sum3 : Sum  Inputs=|-+
  Vector Concatenate : Concatenate  NumInputs=4
  Vector Concatenate1 : Concatenate  NumInputs=4
  "control input " : Outport
  tag scope: e1=global
  wires:
  Vector Concatenate/1 -> Sum/1  "reference signal"
  From Workspace3/1 -> Vector Concatenate/2
  From Workspace2/1 -> Vector Concatenate/3
  From Workspace4/1 -> Vector Concatenate/4
  Sum1/1 -> "control input "/1  "u"
  From Workspace1/1 -> Vector Concatenate/1
  Sum/1 -> Scope1/1, Feedback gain/1  "error"
  Vector Concatenate1/1 -> Sum/2  "real signals"
  [qw1] -> Vector Concatenate1/1
  [q1] -> Scope/1, Vector Concatenate1/3
  [dqw1] -> Vector Concatenate1/2
  [dq1] -> Vector Concatenate1/4
  Feedback gain/1 -> Sum1/2
  From Workspace/1 -> Sum1/1  "feedforward action"
  From Workspace5/1 -> Sum3/1
  [q1] -> Sum3/2
  Sum3/1 -> [e1]

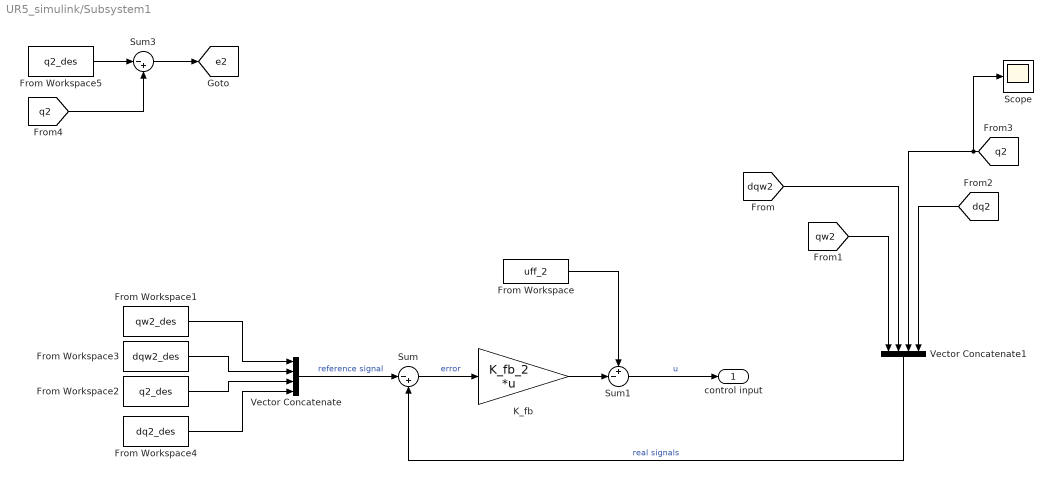
== system UR5_simulink/Subsystem1 ==
  From Workspace : FromWorkspace  VariableName=uff_2
  From Workspace1 : FromWorkspace  VariableName=qw2_des
  From Workspace2 : FromWorkspace  VariableName=q2_des
  From Workspace3 : FromWorkspace  VariableName=dqw2_des
  From Workspace4 : FromWorkspace  VariableName=dq2_des
  From Workspace5 : FromWorkspace  VariableName=q2_des
  K_fb : Gain  Gain=K_fb_2  Multiplication=Matrix(K*u) (u vector)
  Scope : Scope
  Sum : Sum  Inputs=|-+
  Sum1 : Sum  Inputs=+-|
  Sum3 : Sum  Inputs=|-+
  Vector Concatenate : Concatenate  NumInputs=4
  Vector Concatenate1 : Concatenate  NumInputs=4
  "control input " : Outport
  tag scope: e2=global
  wires:
  Vector Concatenate/1 -> Sum/1  "reference signal"
  From Workspace3/1 -> Vector Concatenate/2
  From Workspace2/1 -> Vector Concatenate/3
  From Workspace4/1 -> Vector Concatenate/4
  Sum1/1 -> "control input "/1  "u"
  From Workspace1/1 -> Vector Concatenate/1
  K_fb/1 -> Sum1/2
  Sum/1 -> K_fb/1  "error"
  Vector Concatenate1/1 -> Sum/2  "real signals"
  [qw2] -> Vector Concatenate1/1
  [q2] -> Scope/1, Vector Concatenate1/3
  [dqw2] -> Vector Concatenate1/2
  [dq2] -> Vector Concatenate1/4
  [q2] -> Sum3/2
  From Workspace5/1 -> Sum3/1
  Sum3/1 -> [e2]
  From Workspace/1 -> Sum1/1

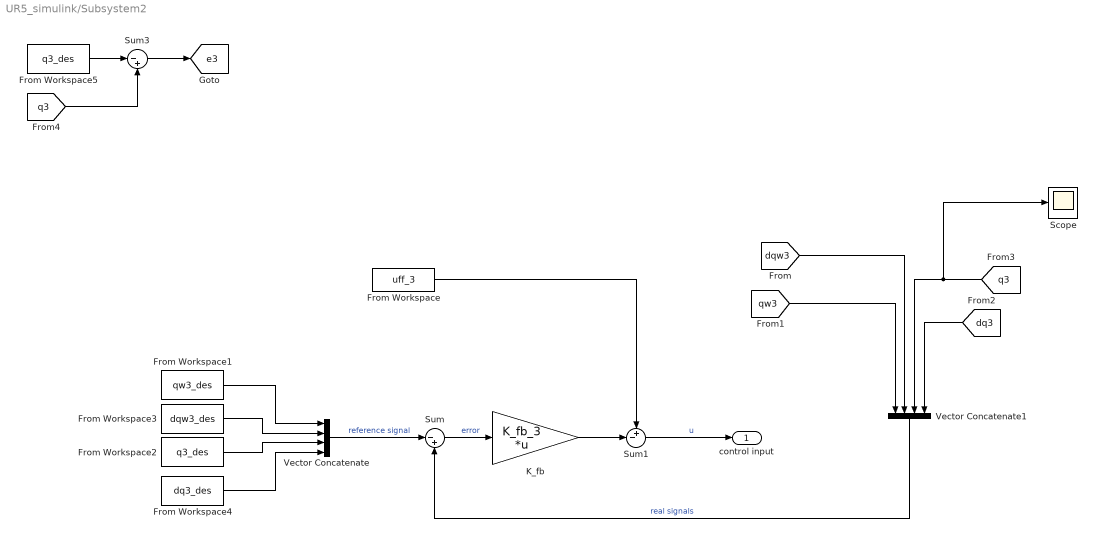
== system UR5_simulink/Subsystem2 ==
  From Workspace : FromWorkspace  VariableName=uff_3
  From Workspace1 : FromWorkspace  VariableName=qw3_des
  From Workspace2 : FromWorkspace  VariableName=q3_des
  From Workspace3 : FromWorkspace  VariableName=dqw3_des
  From Workspace4 : FromWorkspace  VariableName=dq3_des
  From Workspace5 : FromWorkspace  VariableName=q3_des
  K_fb : Gain  Gain=K_fb_3  Multiplication=Matrix(K*u) (u vector)
  Scope : Scope
  Sum : Sum  Inputs=|-+
  Sum1 : Sum  Inputs=+-|
  Sum3 : Sum  Inputs=|-+
  Vector Concatenate : Concatenate  NumInputs=4
  Vector Concatenate1 : Concatenate  NumInputs=4
  "control input " : Outport
  tag scope: e3=global
  wires:
  Vector Concatenate/1 -> Sum/1  "reference signal"
  From Workspace3/1 -> Vector Concatenate/2
  From Workspace2/1 -> Vector Concatenate/3
  From Workspace4/1 -> Vector Concatenate/4
  Sum1/1 -> "control input "/1  "u"
  From Workspace1/1 -> Vector Concatenate/1
  K_fb/1 -> Sum1/2
  Sum/1 -> K_fb/1  "error"
  Vector Concatenate1/1 -> Sum/2  "real signals"
  [qw3] -> Vector Concatenate1/1
  [q3] -> Scope/1, Vector Concatenate1/3
  [dqw3] -> Vector Concatenate1/2
  [dq3] -> Vector Concatenate1/4
  [q3] -> Sum3/2
  From Workspace5/1 -> Sum3/1
  Sum3/1 -> [e3]
  From Workspace/1 -> Sum1/1

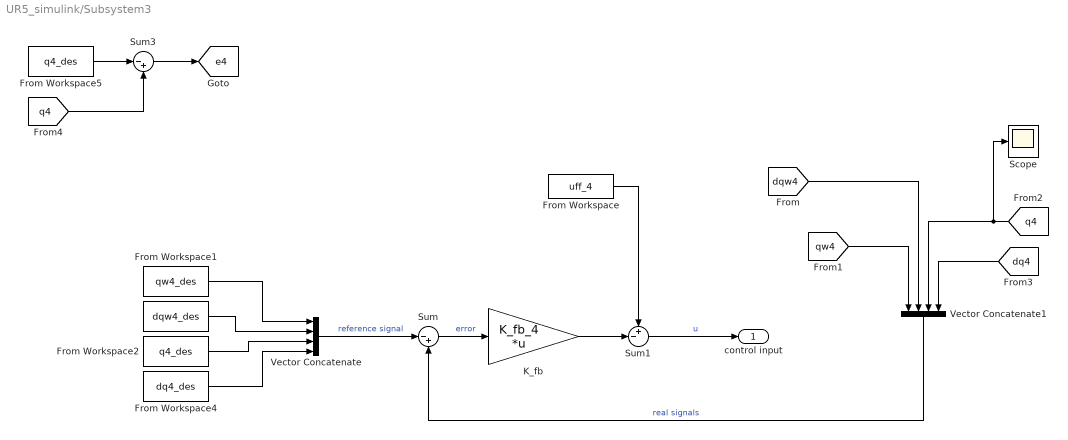
== system UR5_simulink/Subsystem3 ==
  " " : FromWorkspace  VariableName=dqw4_des
  From Workspace : FromWorkspace  VariableName=uff_4
  From Workspace1 : FromWorkspace  VariableName=qw4_des
  From Workspace2 : FromWorkspace  VariableName=q4_des
  From Workspace4 : FromWorkspace  VariableName=dq4_des
  From Workspace5 : FromWorkspace  VariableName=q4_des
  K_fb : Gain  Gain=K_fb_4  Multiplication=Matrix(K*u) (u vector)
  Scope : Scope
  Sum : Sum  Inputs=|-+
  Sum1 : Sum  Inputs=+-|
  Sum3 : Sum  Inputs=|-+
  Vector Concatenate : Concatenate  NumInputs=4
  Vector Concatenate1 : Concatenate  NumInputs=4
  "control input " : Outport
  tag scope: e4=global
  wires:
  Vector Concatenate/1 -> Sum/1  "reference signal"
  " "/1 -> Vector Concatenate/2
  From Workspace2/1 -> Vector Concatenate/3
  From Workspace4/1 -> Vector Concatenate/4
  Sum1/1 -> "control input "/1  "u"
  From Workspace1/1 -> Vector Concatenate/1
  K_fb/1 -> Sum1/2
  Sum/1 -> K_fb/1  "error"
  Vector Concatenate1/1 -> Sum/2  "real signals"
  [qw4] -> Vector Concatenate1/1
  [q4] -> Scope/1, Vector Concatenate1/3
  [dqw4] -> Vector Concatenate1/2
  [dq4] -> Vector Concatenate1/4
  [q4] -> Sum3/2
  From Workspace5/1 -> Sum3/1
  Sum3/1 -> [e4]
  From Workspace/1 -> Sum1/1

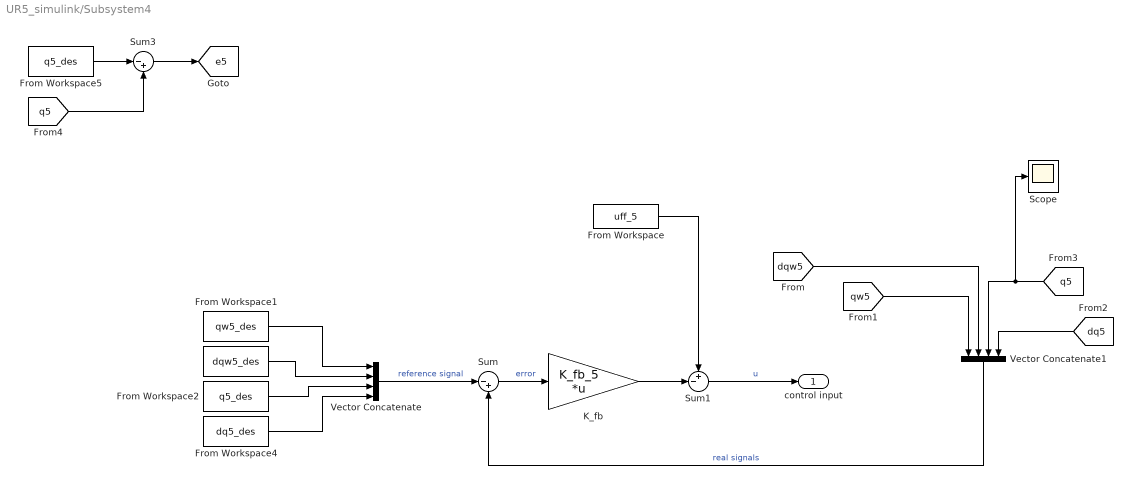
== system UR5_simulink/Subsystem4 ==
  " " : FromWorkspace  VariableName=dqw5_des
  From Workspace : FromWorkspace  VariableName=uff_5
  From Workspace1 : FromWorkspace  VariableName=qw5_des
  From Workspace2 : FromWorkspace  VariableName=q5_des
  From Workspace4 : FromWorkspace  VariableName=dq5_des
  From Workspace5 : FromWorkspace  VariableName=q5_des
  K_fb : Gain  Gain=K_fb_5  Multiplication=Matrix(K*u) (u vector)
  Scope : Scope
  Sum : Sum  Inputs=|-+
  Sum1 : Sum  Inputs=+-|
  Sum3 : Sum  Inputs=|-+
  Vector Concatenate : Concatenate  NumInputs=4
  Vector Concatenate1 : Concatenate  NumInputs=4
  "control input " : Outport
  tag scope: e5=global
  wires:
  Vector Concatenate/1 -> Sum/1  "reference signal"
  " "/1 -> Vector Concatenate/2
  From Workspace2/1 -> Vector Concatenate/3
  From Workspace4/1 -> Vector Concatenate/4
  Sum1/1 -> "control input "/1  "u"
  From Workspace1/1 -> Vector Concatenate/1
  K_fb/1 -> Sum1/2
  Sum/1 -> K_fb/1  "error"
  Vector Concatenate1/1 -> Sum/2  "real signals"
  [qw5] -> Vector Concatenate1/1
  [q5] -> Scope/1, Vector Concatenate1/3
  [dqw5] -> Vector Concatenate1/2
  [dq5] -> Vector Concatenate1/4
  [q5] -> Sum3/2
  From Workspace5/1 -> Sum3/1
  Sum3/1 -> [e5]
  From Workspace/1 -> Sum1/1

== system UR5_simulink/Subsystem5 ==
  " " : FromWorkspace  VariableName=dqw6_des
  From Workspace : FromWorkspace  VariableName=uff_6
  From Workspace1 : FromWorkspace  VariableName=qw6_des
  From Workspace2 : FromWorkspace  VariableName=q6_des
  From Workspace4 : FromWorkspace  VariableName=dq6_des
  From Workspace5 : FromWorkspace  VariableName=q6_des
  K_fb : Gain  Gain=K_fb_6  Multiplication=Matrix(K*u) (u vector)
  Scope : Scope
  Sum : Sum  Inputs=|-+
  Sum1 : Sum  Inputs=+-|
  Sum3 : Sum  Inputs=|-+
  Vector Concatenate : Concatenate  NumInputs=4
  Vector Concatenate1 : Concatenate  NumInputs=4
  "control input " : Outport
  tag scope: e6=global
  wires:
  Vector Concatenate/1 -> Sum/1  "reference signal"
  " "/1 -> Vector Concatenate/2
  From Workspace2/1 -> Vector Concatenate/3
  From Workspace4/1 -> Vector Concatenate/4
  Sum1/1 -> "control input "/1  "u"
  From Workspace1/1 -> Vector Concatenate/1
  K_fb/1 -> Sum1/2
  Sum/1 -> K_fb/1  "error"
  Vector Concatenate1/1 -> Sum/2  "real signals"
  [qw6] -> Vector Concatenate1/1
  [q6] -> Scope/1, Vector Concatenate1/3
  [dqw6] -> Vector Concatenate1/2
  [dq6] -> Vector Concatenate1/4
  [q6] -> Sum3/2
  From Workspace5/1 -> Sum3/1
  Sum3/1 -> [e6]
  From Workspace/1 -> Sum1/1

== system UR5_simulink/HFUS14_4/Custom Spring ==
  Rotational Spring (Custom) of HFUS 14 : MyComponent_lib/Rotational Spring (Custom) of HFUS 14  K_1=4.7 * (10 ^ 3) N*m/rad  K_2=6.1 * (10 ^ 3) N*m/rad  K_3=7.1 * (10 ^ 3) N*m/rad  T_1=2 N*m  T_2=6.9 N*m  b_2=0.596 N*m  b_3=1.825 N*m  phi_1=4.255 * (10 ^ (-4)) rad  phi_2=1.229 * (10 ^ (-3)) rad  w_specify=off  w_priority=None  w=0 rad/s  w_nominal_specify=off  w_nominal_unit=rad/s  w_nominal_value=1  t_specify=off  t_priority=None  t=0 N*m  t_nominal_specify=off  t_nominal_unit=N*m  t_nominal_value=1  phi_specify=off  phi_priority=High  phi=0 rad  phi_nominal_specify=off  phi_nominal_unit=rad  phi_nominal_value=1
      settings: InternalSimscapePortConfiguration="{\"Bottom\":[],\"Left\":[{\"id\":\"R\",\"label\":\"R\",\"type\":\"foundation.mechanical.rotational.rotational\"}],\"Right\":[{\"id\":\"C\",\"label\":\"C\",\"type\":\"foundation.mechanical.rotational.rotational\"}],\"Top\":[]}"
  Conn1 : PMIOPort  Side=Left
  Conn2 : PMIOPort  Port=2  Side=Right
  connections:
  Conn2/RConn1 -- Rotational Spring (Custom) of HFUS 14/RConn1
  Rotational Spring (Custom) of HFUS 14/LConn1 -- Conn1/RConn1

== system UR5_simulink/HFUS14_5/Custom Spring ==
  Rotational Spring (Custom) of HFUS 14 : MyComponent_lib/Rotational Spring (Custom) of HFUS 14  K_1=4.7 * (10 ^ 3) N*m/rad  K_2=6.1 * (10 ^ 3) N*m/rad  K_3=7.1 * (10 ^ 3) N*m/rad  T_1=2 N*m  T_2=6.9 N*m  b_2=0.596 N*m  b_3=1.825 N*m  phi_1=4.255 * (10 ^ (-4)) rad  phi_2=1.229 * (10 ^ (-3)) rad  w_specify=off  w_priority=None  w=0 rad/s  w_nominal_specify=off  w_nominal_unit=rad/s  w_nominal_value=1  t_specify=off  t_priority=None  t=0 N*m  t_nominal_specify=off  t_nominal_unit=N*m  t_nominal_value=1  phi_specify=off  phi_priority=High  phi=0 rad  phi_nominal_specify=off  phi_nominal_unit=rad  phi_nominal_value=1
      settings: InternalSimscapePortConfiguration="{\"Bottom\":[],\"Left\":[{\"id\":\"R\",\"label\":\"R\",\"type\":\"foundation.mechanical.rotational.rotational\"}],\"Right\":[{\"id\":\"C\",\"label\":\"C\",\"type\":\"foundation.mechanical.rotational.rotational\"}],\"Top\":[]}"
  Conn1 : PMIOPort  Side=Left
  Conn2 : PMIOPort  Port=2  Side=Right
  connections:
  Conn2/RConn1 -- Rotational Spring (Custom) of HFUS 14/RConn1
  Rotational Spring (Custom) of HFUS 14/LConn1 -- Conn1/RConn1

== system UR5_simulink/HFUS14_6/Custom Spring1 ==
  Rotational Spring (Custom) of HFUS 14 : MyComponent_lib/Rotational Spring (Custom) of HFUS 14  K_1=4.7 * (10 ^ 3) N*m/rad  K_2=6.1 * (10 ^ 3) N*m/rad  K_3=7.1 * (10 ^ 3) N*m/rad  T_1=2 N*m  T_2=6.9 N*m  b_2=0.596 N*m  b_3=1.825 N*m  phi_1=4.255 * (10 ^ (-4)) rad  phi_2=1.229 * (10 ^ (-3)) rad  w_specify=off  w_priority=None  w=0 rad/s  w_nominal_specify=off  w_nominal_unit=rad/s  w_nominal_value=1  t_specify=off  t_priority=None  t=0 N*m  t_nominal_specify=off  t_nominal_unit=N*m  t_nominal_value=1  phi_specify=off  phi_priority=High  phi=0 rad  phi_nominal_specify=off  phi_nominal_unit=rad  phi_nominal_value=1
      settings: InternalSimscapePortConfiguration="{\"Bottom\":[],\"Left\":[{\"id\":\"R\",\"label\":\"R\",\"type\":\"foundation.mechanical.rotational.rotational\"}],\"Right\":[{\"id\":\"C\",\"label\":\"C\",\"type\":\"foundation.mechanical.rotational.rotational\"}],\"Top\":[]}"
  Conn1 : PMIOPort  Side=Left
  Conn2 : PMIOPort  Port=2  Side=Right
  connections:
  Conn2/RConn1 -- Rotational Spring (Custom) of HFUS 14/RConn1
  Rotational Spring (Custom) of HFUS 14/LConn1 -- Conn1/RConn1

== system UR5_simulink/HFUS20_1/Custom Spring ==
  customSpring20 : MyComponent_lib/customSpring20  K_1=16 * (10 ^ 3) N*m/rad  K_2=25 * (10 ^ 3) N*m/rad  K_3=29 * (10 ^ 3) N*m/rad  T_1=7 N*m  T_2=25 N*m  b_2=3.9375 N*m  b_3=8.5675 N*m  phi_1=4.375 * (10 ^ (-4)) rad  phi_2=1.1575 * (10 ^ (-3)) rad  w_specify=off  w_priority=None  w=0 rad/s  w_nominal_specify=off  w_nominal_unit=rad/s  w_nominal_value=1  t_specify=off  t_priority=None  t=0 N*m  t_nominal_specify=off  t_nominal_unit=N*m  t_nominal_value=1  phi_specify=off  phi_priority=High  phi=0 rad  phi_nominal_specify=off  phi_nominal_unit=rad  phi_nominal_value=1
      settings: InternalSimscapePortConfiguration="{\"Bottom\":[],\"Left\":[{\"id\":\"R\",\"label\":\"R\",\"type\":\"foundation.mechanical.rotational.rotational\"}],\"Right\":[{\"id\":\"C\",\"label\":\"C\",\"type\":\"foundation.mechanical.rotational.rotational\"}],\"Top\":[]}"
  Conn1 : PMIOPort  Side=Left
  Conn2 : PMIOPort  Port=2  Side=Right
  connections:
  customSpring20/RConn1 -- Conn2/RConn1
  customSpring20/LConn1 -- Conn1/RConn1

== system UR5_simulink/HFUS20_2/Custom Spring ==
  customSpring20 : MyComponent_lib/customSpring20  K_1=16 * (10 ^ 3) N*m/rad  K_2=25 * (10 ^ 3) N*m/rad  K_3=29 * (10 ^ 3) N*m/rad  T_1=7 N*m  T_2=25 N*m  b_2=3.9375 N*m  b_3=8.5675 N*m  phi_1=4.375 * (10 ^ (-4)) rad  phi_2=1.1575 * (10 ^ (-3)) rad  w_specify=off  w_priority=None  w=0 rad/s  w_nominal_specify=off  w_nominal_unit=rad/s  w_nominal_value=1  t_specify=off  t_priority=None  t=0 N*m  t_nominal_specify=off  t_nominal_unit=N*m  t_nominal_value=1  phi_specify=off  phi_priority=High  phi=0 rad  phi_nominal_specify=off  phi_nominal_unit=rad  phi_nominal_value=1
      settings: InternalSimscapePortConfiguration="{\"Bottom\":[],\"Left\":[{\"id\":\"R\",\"label\":\"R\",\"type\":\"foundation.mechanical.rotational.rotational\"}],\"Right\":[{\"id\":\"C\",\"label\":\"C\",\"type\":\"foundation.mechanical.rotational.rotational\"}],\"Top\":[]}"
  Conn1 : PMIOPort  Side=Left
  Conn2 : PMIOPort  Port=2  Side=Right
  connections:
  customSpring20/RConn1 -- Conn2/RConn1
  Conn1/RConn1 -- customSpring20/LConn1

== system UR5_simulink/HFUS20_3/Custom Spring ==
  customSpring20 : MyComponent_lib/customSpring20  K_1=16 * (10 ^ 3) N*m/rad  K_2=25 * (10 ^ 3) N*m/rad  K_3=29 * (10 ^ 3) N*m/rad  T_1=7 N*m  T_2=25 N*m  b_2=3.9375 N*m  b_3=8.5675 N*m  phi_1=4.375 * (10 ^ (-4)) rad  phi_2=1.1575 * (10 ^ (-3)) rad  w_specify=off  w_priority=None  w=0 rad/s  w_nominal_specify=off  w_nominal_unit=rad/s  w_nominal_value=1  t_specify=off  t_priority=None  t=0 N*m  t_nominal_specify=off  t_nominal_unit=N*m  t_nominal_value=1  phi_specify=off  phi_priority=High  phi=0 rad  phi_nominal_specify=off  phi_nominal_unit=rad  phi_nominal_value=1
      settings: InternalSimscapePortConfiguration="{\"Bottom\":[],\"Left\":[{\"id\":\"R\",\"label\":\"R\",\"type\":\"foundation.mechanical.rotational.rotational\"}],\"Right\":[{\"id\":\"C\",\"label\":\"C\",\"type\":\"foundation.mechanical.rotational.rotational\"}],\"Top\":[]}"
  Conn1 : PMIOPort  Side=Left
  Conn2 : PMIOPort  Port=2  Side=Right
  connections:
  customSpring20/LConn1 -- Conn1/RConn1
  Conn2/RConn1 -- customSpring20/RConn1
